simulink subsystem "DrivePattern_refsub"  (R2023a)
settings: Solver=VariableStepAuto  StartTime=0.0  StopTime=10.0  RelTol=1e-3
undefined symbols (not defined in the file): drivePatternFromWorkspace
libraries: autolibshared x1
settings Model: Creator=isaacito  LastModifiedBy=isaacito
settings SolverCC: AlgebraicLoopSolver=TrustRegion
settings DebuggingCC: UnconnectedInputMsg=warning  UnconnectedOutputMsg=warning  UnconnectedLineMsg=warning
settings ModelReferenceCC: EnableRefExpFcnMdlSchedulingChecks=on
settings RTWCC: DLArmComputeVersion=19.05

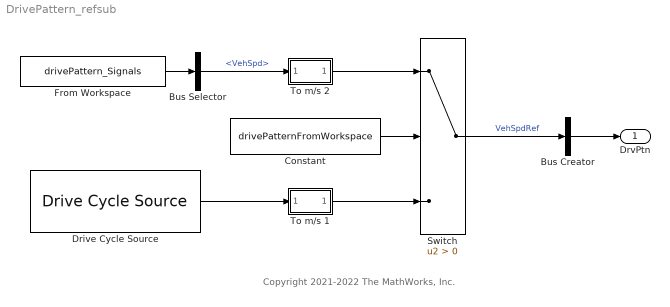
== system DrivePattern_refsub ==
  note: Copyright 2021-2022 The MathWorks, Inc.
  Bus Creator : BusCreator  Inputs=1
  Bus Selector : BusSelector  OutputSignals=VehSpd
  Constant : Constant  Value=drivePatternFromWorkspace
  Drive Cycle Source : autolibshared/Drive Cycle Source  cycleVar=FTP75  fileVar=cycleFTP75.mat  tfinal="2474  seconds"  cycleRepeat=off  outAccPort=off  outGearPort=off  gearList=No gear data  t_wot1=5  xdot_woto=0  xdot_wot1=30  t_wot2=20  xdot_wot2=0  t_wotend=30  srcUnit=m/s  outUnit=mph  srcAccUnit=m/s/s  outAccUnit=m/s^2  dt=0  aMode=1  faultOption=off  velBnd=2  velBndUnit=mph  inUnit=m/s  timeBnd=1  failOption=off  stopSim=off  maxFaultCnt=10  maxFaultTime=2  maxTotFaultTime=15  traceOption=off  dtTrace=1  traceWindow=10  lastDCname=FTP75  lastOutUnit=mph  lastDT=0  lastTB=1  lastSB=2  forceCalcBound=off
  From Workspace : FromWorkspace  VariableName=drivePattern_Signals  OutDataTypeStr=Bus: drivePattern_Bus  OutputAfterFinalValue=Holding final value
      settings: AttributesFormatString=|
      | %<OutDataTypeStr>
      | Interpolate: %<Interpolate>
  Switch : Switch  Criteria=u2 > Threshold  SaturateOnIntegerOverflow=off  InputSameDT=off
  To m/s 1 : Subsystem
  To m/s 2 : Subsystem
  DrvPtn : Outport
  wires:
  Switch/1 -> Bus Creator/1  "VehSpdRef"
  To m/s 1/1(Out1) -> Switch/3
  Drive Cycle Source/1 -> To m/s 1/1(In1)
  To m/s 2/1(Out1) -> Switch/1
  Bus Selector/1 -> To m/s 2/1(In1)  "<VehSpd>"
  Bus Creator/1 -> DrvPtn/1
  From Workspace/1 -> Bus Selector/1
  Constant/1 -> Switch/2

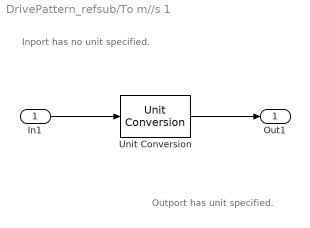
== system DrivePattern_refsub/To m//s 1 ==
  note: Inport has no unit specified.
  note: Outport has unit specified.
  In1 : Inport
  Unit Conversion : UnitConversion
  Out1 : Outport  Unit=m/s
  wires:
  Unit Conversion/1 -> Out1/1
  In1/1 -> Unit Conversion/1

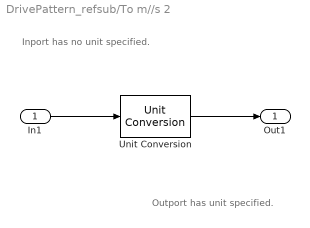
== system DrivePattern_refsub/To m//s 2 ==
  note: Inport has no unit specified.
  note: Outport has unit specified.
  In1 : Inport
  Unit Conversion : UnitConversion
  Out1 : Outport  Unit=m/s
  wires:
  Unit Conversion/1 -> Out1/1
  In1/1 -> Unit Conversion/1
